simulink model "hw_microgrids1_with_sctrl"  (R2024b)
settings: Solver=ode45  StartTime=0.0  StopTime=simu.endTime  MaxStep=simu.maxStepSize  RelTol=1e-3
undefined symbols (not defined in the file or in its folder): es, mg, wt
libraries: simulink x1
settings Model: Creator=tedbrekken  LastModifiedBy=kerrychen
settings RTWCC: GPUComputeCapability=3.5

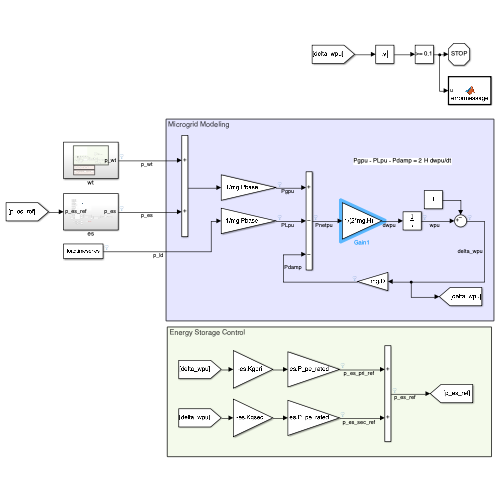
[thumbnail: Simulink's stored preview of the top-level diagram]
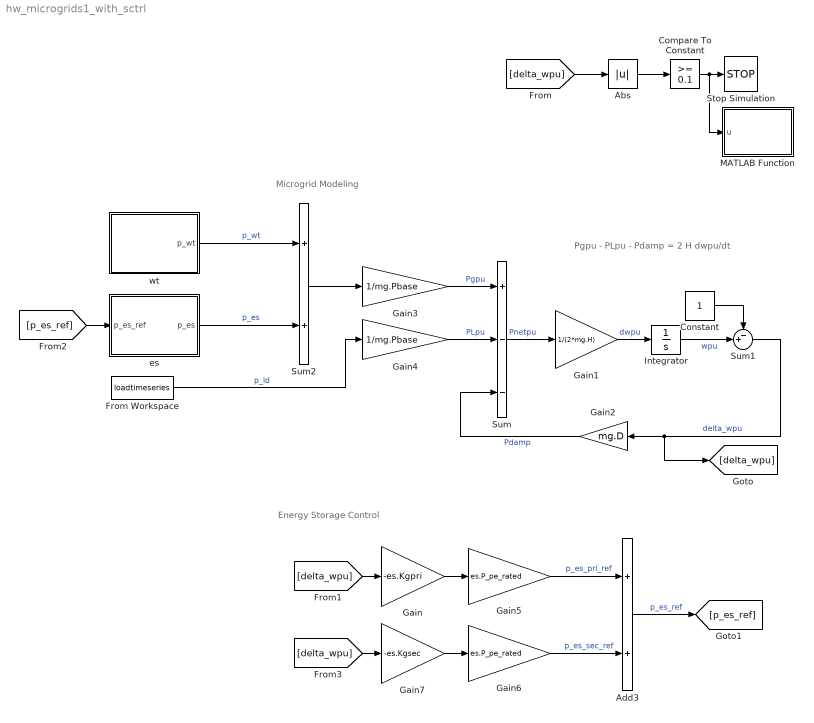
== system hw_microgrids1_with_sctrl ==
  note: Energy Storage Control
  note: Microgrid Modeling
  note: Pgpu - PLpu - Pdamp = 2 H dwpu/dt
  Abs : Abs  SaturateOnIntegerOverflow=off
  Add3 : Sum
  Compare To Constant : simulink/Logic and Bit Operations/Compare To Constant  relop=>=  const=0.1  OutDataTypeStr=boolean
  Constant : Constant
  From Workspace : FromWorkspace  VariableName=loadtimeseries  OutputAfterFinalValue=Setting to zero
  Gain : Gain  Gain=-es.Kgpri
  Gain1 : Gain  Gain=1/(2*mg.H)
  Gain2 : Gain  Gain=mg.D
  Gain3 : Gain  Gain=1/mg.Pbase
  Gain4 : Gain  Gain=1/mg.Pbase
  Gain5 : Gain  Gain=es.P_pe_rated
  Gain6 : Gain  Gain=es.P_pe_rated
  Gain7 : Gain  Gain=-es.Kgsec
  Integrator : Integrator  InitialCondition=mg.wpu_0
  MATLAB Function : MATLAB Function  TreatAsAtomicUnit=on
  Stop Simulation : Stop
  Sum : Sum  Inputs=+--
  Sum1 : Sum  Inputs=-+|
  Sum2 : Sum
  es : Subsystem
  wt : Subsystem
  wires:
  Sum/1 -> Gain1/1  "Pnetpu"
  Gain1/1 -> Integrator/1  "dwpu"
  Integrator/1 -> Sum1/2  "wpu"
  Constant/1 -> Sum1/1
  Sum1/1 -> [delta_wpu], Gain2/1  "delta_wpu"
  Gain2/1 -> Sum/3  "Pdamp"
  Gain3/1 -> Sum/1  "Pgpu"
  Gain4/1 -> Sum/2  "PLpu"
  wt/1(p_wt) -> Sum2/1  "p_wt"
  es/1(p_es) -> Sum2/2  "p_es"
  Sum2/1 -> Gain3/1
  From Workspace/1 -> Gain4/1  "p_ld"
  [delta_wpu] -> Abs/1
  Abs/1 -> Compare To Constant/1
  Compare To Constant/1 -> MATLAB Function/1(u), Stop Simulation/1
  [p_es_ref] -> es/1(p_es_ref)
  [delta_wpu] -> Gain/1
  Gain/1 -> Gain5/1
  Gain5/1 -> Add3/1  "p_es_pri_ref"
  Gain6/1 -> Add3/2  "p_es_sec_ref"
  Add3/1 -> [p_es_ref]  "p_es_ref"
  Gain7/1 -> Gain6/1
  [delta_wpu] -> Gain7/1

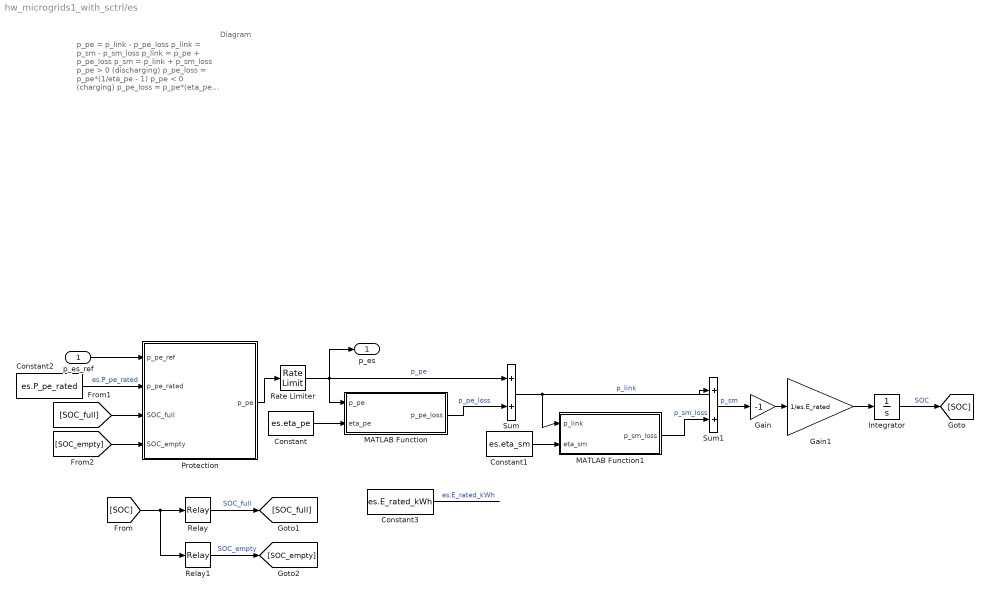
== system hw_microgrids1_with_sctrl/es ==
  note: Diagram
  note: p_pe = p_link - p_pe_loss
      | p_link = p_sm - p_sm_loss
      |
      | p_link = p_pe + p_pe_loss
      | p_sm = p_link + p_sm_loss
      |
      | p_pe > 0 (discharging)
      | p_pe_loss = p_pe*(1/eta_pe - 1)
      |
      | p_pe < 0 (charging)
      | p_pe_loss = p_pe*(eta_pe - 1)
      |
      | p_link > 0 (discharging)
      | p_sm_loss = p_link*(1/eta_sm - 1)
      |
      | p_link < 0 (charging)
      | p_sm_loss = p_link*(eta_sm - 1)
      |
      | e_sm = - int(p_sm)
      |
      | SOC = e_sm / es.E_rated
      |
      | if p_pe_ref > p_pe_upper
      | p_pe = p_pe_upper
      |
      | if p_pe_ref < p_pe_lower
      | p_pe = p_pe_lower
      |
      | if SOC >= 1
      | p_pe_lower = 0
      |
      | if SOC <= 0
      | p_pe_upper = 0
  p_es_ref : Inport
  Constant : Constant  Value=es.eta_pe
  Constant1 : Constant  Value=es.eta_sm
  Constant2 : Constant  Value=es.P_pe_rated
  Constant3 : Constant  Value=es.E_rated_kWh
  Gain : Gain  Gain=-1
  Gain1 : Gain  Gain=1/es.E_rated
  Integrator : Integrator  InitialCondition=es.SOC_0
  MATLAB Function : MATLAB Function  TreatAsAtomicUnit=on
  MATLAB Function1 : MATLAB Function  TreatAsAtomicUnit=on
  Protection : MATLAB Function  TreatAsAtomicUnit=on
  Rate Limiter : RateLimiter  RisingSlewLimit=es.P_pe_slew_upper  FallingSlewLimit=es.P_pe_slew_lower  SampleTimeMode=inherited
  Relay : Relay  OnSwitchValue=1.01  OffSwitchValue=0.99
  Relay1 : Relay  OnSwitchValue=0.01  OffSwitchValue=-0.01  OnOutputValue=0  OffOutputValue=1
  Sum : Sum
  Sum1 : Sum
  p_es : Outport
  wires:
  [SOC_empty] -> Protection/4(SOC_empty)
  Relay1/1 -> [SOC_empty]  "SOC_empty"
  [SOC_full] -> Protection/3(SOC_full)
  Gain1/1 -> Integrator/1
  Relay/1 -> [SOC_full]  "SOC_full"
  Gain/1 -> Gain1/1
  Constant/1 -> MATLAB Function/2(eta_pe)
  [SOC] -> Relay1/1, Relay/1
  Constant2/1 -> Protection/2(p_pe_rated)  "es.P_pe_rated"
  MATLAB Function/1(p_pe_loss) -> Sum/2  "p_pe_loss"
  Constant1/1 -> MATLAB Function1/2(eta_sm)
  p_es_ref/1 -> Protection/1(p_pe_ref)
  MATLAB Function1/1(p_sm_loss) -> Sum1/2  "p_sm_loss"
  Integrator/1 -> [SOC]  "SOC"
  Sum1/1 -> Gain/1  "p_sm"
  Sum/1 -> MATLAB Function1/1(p_link), Sum1/1  "p_link"
  Protection/1(p_pe) -> Rate Limiter/1
  Rate Limiter/1 -> p_es/1, Sum/1, MATLAB Function/1(p_pe)  "p_pe"
  Constant3/1 -> ?  "es.E_rated_kWh"

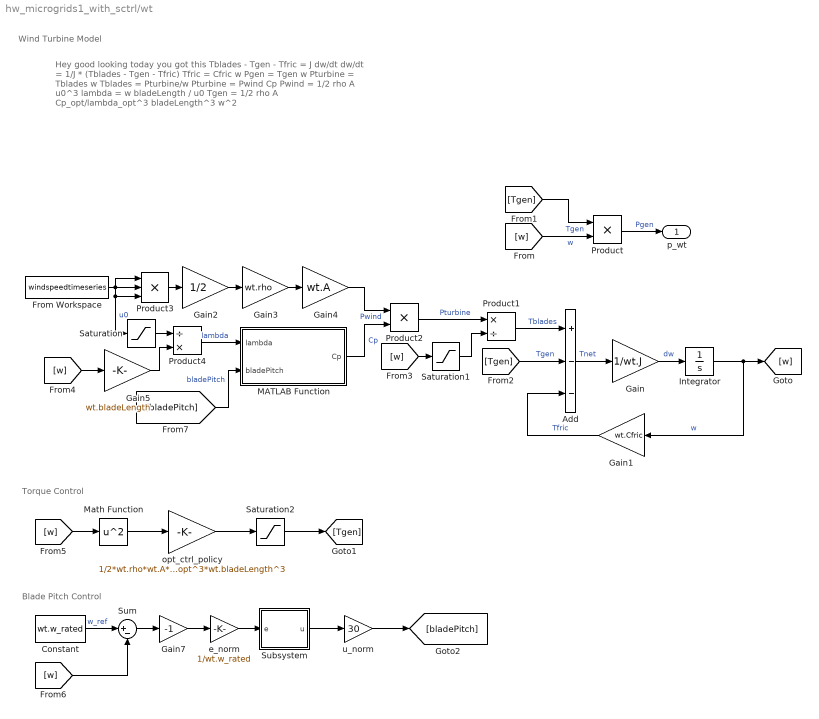
== system hw_microgrids1_with_sctrl/wt ==
  note: Blade Pitch Control
  note: Wind Turbine Model
  note: Hey good looking today you got this
      |
      | Tblades - Tgen - Tfric = J dw/dt
      | dw/dt = 1/J * (Tblades - Tgen - Tfric)
      | Tfric = Cfric w
      |
      | Pgen = Tgen w
      |
      | Pturbine = Tblades w
      | Tblades = Pturbine/w
      |
      | Pturbine = Pwind Cp
      |
      | Pwind = 1/2 rho A u0^3
      |
      | lambda = w bladeLength / u0
      |
      | Tgen = 1/2 rho A Cp_opt/lambda_opt^3 bladeLength^3 w^2
  note: Torque Control
  Add : Sum  Inputs=+--
  Constant : Constant  Value=wt.w_rated
  From Workspace : FromWorkspace  VariableName=windspeedtimeseries
  Gain : Gain  Gain=1/wt.J
  Gain1 : Gain  Gain=wt.Cfric
  Gain2 : Gain  Gain=1/2
  Gain3 : Gain  Gain=wt.rho
  Gain4 : Gain  Gain=wt.A
  Gain5 : Gain  Gain=wt.bladeLength
  Gain7 : Gain  Gain=-1
  Integrator : Integrator  InitialCondition=wt.w_0
  MATLAB Function : MATLAB Function  TreatAsAtomicUnit=on
  Math Function : Math  Operator=square
  Product : Product
  Product1 : Product  Inputs=*/
  Product2 : Product
  Product3 : Product  Inputs=3
  Product4 : Product  Inputs=/*
  Saturation : Saturate  UpperLimit=inf  LowerLimit=1e-3
  Saturation1 : Saturate  UpperLimit=inf  LowerLimit=1e-3
  Saturation2 : Saturate  UpperLimit=wt.Tgen_rated  LowerLimit=0
  Subsystem : Subsystem  mask{kp=wt.pitchctrl.kp, ki=wt.pitchctrl.ki, upperLimit=wt.pitchctrl.upperLimit, lowerLimit=wt.pitchctrl.lowerLimit}
      mask prompts: kp "Proportional gain"; ki "Integral gain"; upperLimit "Upper limit"; lowerLimit "Lower limit"
  Sum : Sum  Inputs=|+-
  e_norm : Gain  Gain=1/wt.w_rated
  opt_ctrl_policy : Gain  Gain=1/2*wt.rho*wt.A*wt.Cp_opt/wt.lambda_opt^3*wt.bladeLength^3
  u_norm : Gain  Gain=30
  p_wt : Outport
  wires:
  Constant/1 -> Sum/1  "w_ref"
  Product1/1 -> Add/1  "Tblades"
  Gain2/1 -> Gain3/1
  [w] -> Saturation1/1
  Gain1/1 -> Add/3  "Tfric"
  u_norm/1 -> [bladePitch]
  Sum/1 -> Gain7/1
  Math Function/1 -> opt_ctrl_policy/1
  Product4/1 -> MATLAB Function/1(lambda)  "lambda"
  Saturation/1 -> Product4/1
  [Tgen] -> Product/1  "Tgen"
  Gain4/1 -> Product2/1  "Pwind"
  e_norm/1 -> Subsystem/1(e)
  Add/1 -> Gain/1  "Tnet"
  [w] -> Math Function/1
  MATLAB Function/1(Cp) -> Product2/2  "Cp"
  Saturation1/1 -> Product1/2
  Saturation2/1 -> [Tgen]
  Gain7/1 -> e_norm/1
  [w] -> Sum/2
  opt_ctrl_policy/1 -> Saturation2/1
  Gain5/1 -> Product4/2
  Product/1 -> p_wt/1  "Pgen"
  Subsystem/1(u) -> u_norm/1
  [w] -> Gain5/1
  Product2/1 -> Product1/1  "Pturbine"
  Integrator/1 -> [w], Gain1/1  "w"
  [w] -> Product/2  "w"
  Product3/1 -> Gain2/1
  Gain3/1 -> Gain4/1
  From Workspace/1 -> Saturation/1, Product3/3, Product3/2, Product3/1  "u0"
  [Tgen] -> Add/2  "Tgen"
  [bladePitch] -> MATLAB Function/2(bladePitch)  "bladePitch"
  Gain/1 -> Integrator/1  "dw"

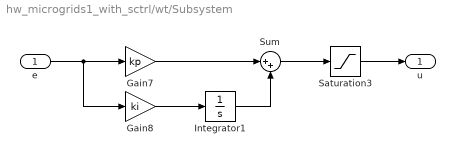
== system hw_microgrids1_with_sctrl/wt/Subsystem ==
  e : Inport
  Gain7 : Gain  Gain=kp
  Gain8 : Gain  Gain=ki
  Integrator1 : Integrator  LimitOutput=on  UpperSaturationLimit=upperLimit  LowerSaturationLimit=lowerLimit
  Saturation3 : Saturate  UpperLimit=upperLimit  LowerLimit=lowerLimit
  Sum : Sum  Inputs=|++
  u : Outport
  wires:
  Integrator1/1 -> Sum/2
  Saturation3/1 -> u/1
  e/1 -> Gain8/1, Gain7/1
  Gain8/1 -> Integrator1/1
  Gain7/1 -> Sum/1
  Sum/1 -> Saturation3/1

== matlab function hw_microgrids1_with_sctrl/es/MATLAB Function ==
  data: p_pe input; p_pe_loss output; eta_pe input
function p_pe_loss = fcn(p_pe,eta_pe)
% p_pe > 0 (discharging)
% p_pe_loss = p_pe*(1/eta_pe - 1)
%
% p_pe < 0 (charging)
% p_pe_loss = p_pe*(eta_pe - 1)

if p_pe > 0
    p_pe_loss = p_pe*(1/eta_pe-1);
elseif p_pe < 0
    p_pe_loss = p_pe*(eta_pe-1);
elseif p_pe == 0
    p_pe_loss = 0;
else
    error("I didnt think of this")
end

== matlab function hw_microgrids1_with_sctrl/wt/MATLAB Function ==
  data: lambda input; Cp output; bladePitch input
function Cp = fcn(lambda,bladePitch)

% https://www.mathworks.com/help/physmod/sps/powersys/ref/windturbine.html

c = [...
    0.5176 ...
    116 ...
    0.4 ...
    5 ...
    21 ...
    0.0068];

if (lambda+0.08*bladePitch) == 0
    lambda = 1e-3;
end

lambdaai = 1/( 1/(lambda+0.08*bladePitch) - 0.035/(bladePitch^3+1) );

Cp = c(1)*(c(2)/lambdaai-c(3)*bladePitch-c(4))*exp(-c(5)/lambdaai) + c(6)*lambda;

== matlab function hw_microgrids1_with_sctrl/es/MATLAB Function1 ==
  data: p_link input; p_sm_loss output; eta_sm input
function p_sm_loss = fcn(p_link,eta_sm)
% p_link > 0 (discharging)
% p_sm_loss = p_link*(1/eta_sm - 1)
%
% p_link < 0 (charging)
% p_sm_loss = p_link*(eta_sm - 1)

if p_link > 0
    p_sm_loss = p_link*(1/eta_sm-1);
elseif p_link < 0
    p_sm_loss = p_link*(eta_sm-1);
elseif p_link == 0
    p_sm_loss = 0;
else
    error("I didnt think of this")
end

== matlab function hw_microgrids1_with_sctrl/es/Protection ==
  data: p_pe_ref input; p_pe output; p_pe_rated input; SOC_full input; SOC_empty input
function p_pe = fcn(p_pe_ref,p_pe_rated,SOC_full,SOC_empty)
% p_pe_upper = p_pe_rated
% p_pe_lower = -p_pe_rated
%
% if SOC >= 1
% p_pe_lower = 0
% 
% if SOC <= 0
% p_pe_upper = 0
%
% if p_pe_ref > p_pe_upper
% p_pe = p_pe_upper
% 
% if p_pe_ref < p_pe_lower
% p_pe = p_pe_lower

p_pe_upper = p_pe_rated; % 10
p_pe_lower = -p_pe_rated; % -10

if SOC_full
    p_pe_lower = 0; % 0
end

if SOC_empty
    p_pe_upper = 0;
end

if p_pe_ref > p_pe_upper
    p_pe = p_pe_upper;
elseif p_pe_ref < p_pe_lower
    p_pe = p_pe_lower;
else
    p_pe = p_pe_ref;
end

== matlab function hw_microgrids1_with_sctrl/MATLAB Function ==
  data: u input
function errormessage(u)

if u == 1
    error("!!!Microgrid exploded due to mismanagement!!!")
end
